simulink model "rotpentemplate"  (R2021b)
settings: Solver=ode45  StartTime=0.0  StopTime=100  RelTol=1e-3  EnableMultiTasking=on
values from neighbouring files (symbols this model uses):
  adingain = cfg.adingain    [hwinit.m]
  adinoffs = cfg.adinoffs    [hwinit.m]
  daoutgain = cfg.daoutgain    [hwinit.m]
  daoutoffs = cfg.daoutoffs    [hwinit.m]
  h = cfg.h    [hwinit.m]    (also in multisine.m = 0.005; prbs_signal.m = 0.001)
libraries: slpidlib x1
settings Model: Creator=rbabuska  LastModifiedBy=tsderksen
settings SolverCC: AlgebraicLoopSolver=TrustRegion
settings DataIOCC: LimitDataPoints=on  SaveFormat=Array  ReturnWorkspaceOutputs=off  SignalLoggingName=sigsOut
settings OptimizationCC: BooleanDataType=off  ExpressionDepthLimit=2147483647  InitFltsAndDblsToZero=on  LifeSpan=inf
settings DebuggingCC: SaveWithParameterizedLinksMsg=none  SignalResolutionControl=TryResolveAllWithWarning  MultiTaskDSMMsg=warning  MultiTaskCondExecSysMsg=none  AllowSymbolicDim=off  StateNameClashWarn=warning  SFUnexpectedBacktrackingDiag=warning  SFNoUnconditionalDefaultTransitionDiag=warning  SFExecutionAtInitializationDiag=none  SFMachineParentedDataDiag=warning  ArithmeticOperatorsInVariantConditions=warning
settings HardwareCC: ProdBitPerPointer=32  ProdBitPerSizeT=32  ProdBitPerPtrDiffT=32  ProdLargestAtomicFloat=None  ProdIntDivRoundTo=Undefined  ProdEndianess=Unspecified  ProdWordSize=32  ProdHWDeviceType=32-bit Generic  TargetUnknown=on
settings ModelReferenceCC: PropagateSignalLabelsOutOfModel=off
settings SFSimCC: SimUseLocalCustomCode=off  CustomCodeUndefinedFunction=UseInterfaceOnly
settings RTWCC: RTWUseLocalCustomCode=off
settings CodeAppCC: StateflowObjectComments=on
settings GRTTargetCC: TargetFcnLib=ansi_tfl_tmw.mat  TargetLangStandard=C89/C90 (ANSI)  CombineOutputUpdateFcns=off  GRTInterface=on
settings ConfigComp: CovMetricSettings=dw  CovSaveCumulativeToWorkspaceVar=on  CovSaveSingleToWorkspaceVar=on  CovExternalEMLEnable=off

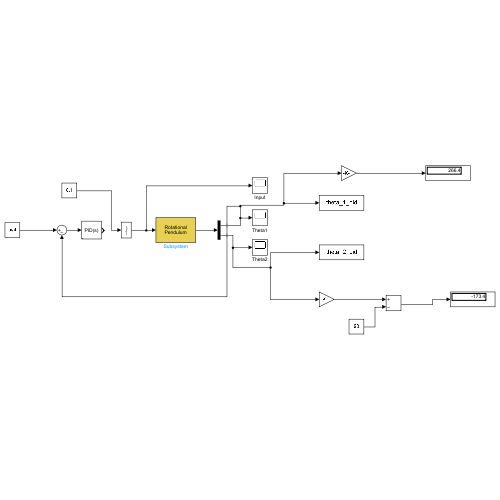
[thumbnail: Simulink's stored preview of the top-level diagram]
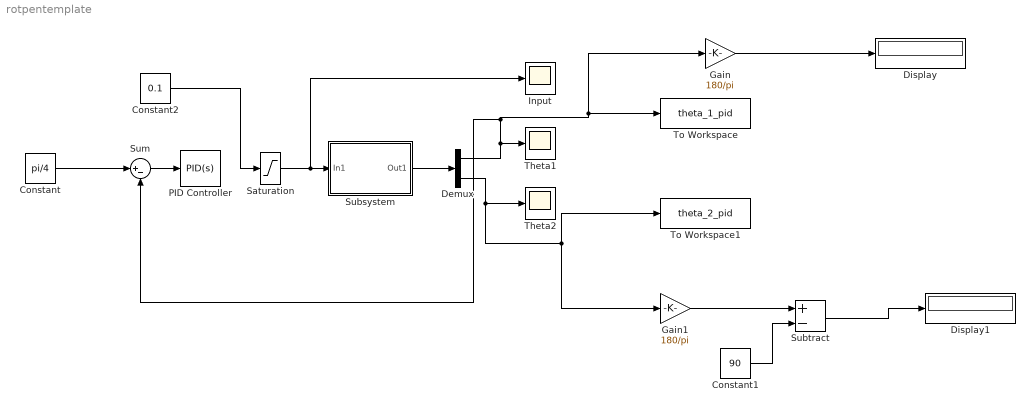
== system rotpentemplate ==
  Constant : Constant  Value=pi/4
  Constant1 : Constant  Value=90
  Constant2 : Constant  Value=0.1
  Demux : Demux  Outputs=2
  Display : Display
  Display1 : Display
  Gain : Gain  Gain=180/pi
  Gain1 : Gain  Gain=180/pi
  Input : Scope
  PID Controller : slpidlib/PID Controller  Controller=PID  Form=Parallel  TimeDomain=Continuous-time  UseExternalTs=off  SampleTime=-1  IntegratorMethod=Forward Euler  FilterMethod=Forward Euler  ControllerParametersSource=internal  P=0.1  I=0.1  D=0  UseFilter=on  N=100  TunerSelectOption=Transfer Function Based (PID Tuner App)  InitialConditionSource=internal  InitialConditionForIntegrator=0  InitialConditionForFilter=0  DifferentiatorICPrevScaledInput=0  ExternalReset=none  TrackingMode=off  Kt=1  LimitOutput=off  SatLimitsSource=internal  UpperSaturationLimit=inf  LowerSaturationLimit=-inf  LinearizeAsGain=on  AntiWindupMode=none  Kb=1  POutMin=[]  POutMax=[]  IOutMin=[]  IOutMax=[]  DOutMin=[]  DOutMax=[]  NOutMin=[]  NOutMax=[]  SumOutMin=[]  SumOutMax=[]  SaturationOutMin=[]  SaturationOutMax=[]  PParamMin=[]  PParamMax=[]  IParamMin=[]  IParamMax=[]  DParamMin=[]  DParamMax=[]  NParamMin=[]  NParamMax=[]  KbParamMin=[]  KbParamMax=[]  KtParamMin=[]  KtParamMax=[]  KbOutMin=[]  KbOutMax=[]  KtOutMin=[]  KtOutMax=[]  IntegratorOutMin=[]  IntegratorOutMax=[]  FilterOutMin=[]  FilterOutMax=[]  SumI1OutMin=[]  SumI1OutMax=[]  SumI2OutMin=[]  SumI2OutMax=[]  SumI3OutMin=[]  SumI3OutMax=[]  SumI4OutMin=[]  SumI4OutMax=[]  SumDOutMin=[]  SumDOutMax=[]  DifferentiatorOutMin=[]  DifferentiatorOutMax=[]  FilterDiffOutCoefMin=[]  FilterDiffOutCoefMax=[]  ReciprocalOutMin=[]  ReciprocalOutMax=[]  SumDenOutMin=[]  SumDenOutMax=[]  SumNumOutMin=[]  SumNumOutMax=[]  DivideOutMin=[]  DivideOutMax=[]  UdiffTsProdOutMin=[]  UdiffTsProdOutMax=[]  NTsProdOutMin=[]  NTsProdOutMax=[]  UintegralTsProdOutMin=[]  UintegralTsProdOutMax=[]  UngainTsProdOutMin=[]  UngainTsProdOutMax=[]  IntegratorContinuousStateAttributes=''  IntegratorStateMustResolveToSignalObject=off  IntegratorRTWStateStorageClass=Auto  FilterContinuousStateAttributes=''  FilterStateMustResolveToSignalObject=off  FilterRTWStateStorageClass=Auto  ParallelPVariant=InternalParameters  IdealPVariant=Disabled  IVariant=InternalParameters  DVariant=InternalParameters  IntegratorVariant=Continuous  SatVariant=Disabled  AWVariant=Passthrough  PCopyVariant=Disabled  TRVariant=Disabled  FdbkBlocksVariant=Forward  IdealPFdbkVariant=Disabled  SatFdbkVariant=Disabled  DerivativeFilterVariant=ContFilter  NVariant=InternalParameters  NCopyVariant=Disabled  FilterICVariant=InternalICsFilter  IntegratorICVariant=InternalICs  ExternalResetVariant=Disabled  TRSumVariant=Passthrough  SumFdbkVariant=Disabled  SumVariant=Sum_PID  TsampFilterVariant=InternalTs  TsampNgainVariant=Passthrough  TsampIntegralVariant=Passthrough  ExternalSaturationOutDataTypeStr=Inherit: Same as second input
  Saturation : Saturate  UpperLimit=1  LowerLimit=-1
  Subsystem : Subsystem
      mask Display: disp('Rotational\nPendulum')
  Subtract : Sum  Inputs=+-
  Sum : Sum  Inputs=|+-
  Theta1 : Scope
  Theta2 : Scope
  To Workspace : ToWorkspace  VariableName=theta_1_pid  SaveFormat=Timeseries  SampleTime=-1
  To Workspace1 : ToWorkspace  VariableName=theta_2_pid  SaveFormat=Timeseries  SampleTime=-1
  wires:
  Saturation/1 -> Subsystem/1(In1), Input/1
  Subsystem/1(Out1) -> Demux/1
  Demux/1 -> Theta1/1, Sum/2, To Workspace/1, Gain/1
  Demux/2 -> Theta2/1, Gain1/1, To Workspace1/1
  Constant1/1 -> Subtract/2
  Subtract/1 -> Display1/1
  Gain1/1 -> Subtract/1
  Gain/1 -> Display/1
  Constant/1 -> Sum/1
  Sum/1 -> PID Controller/1
  Constant2/1 -> Saturation/1

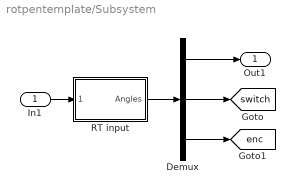
== system rotpentemplate/Subsystem ==
  In1 : Inport
  Demux : Demux  Outputs=[2 4 1]
  RT input : Subsystem  mask{Ts=h, channels=[6 7]}
      mask prompts: Ts "Sample time [s]:"; channels "Channels to read (e.g., [6 7])"
      mask init:
      | hwinit;
      | 
      | % initialize FPGA
      | fugihandle = fugiboard('Open', 'Pendulum1');
      | fugihandle.WatchdogTimeout = 0.5;
      | fugiboard('SetParams', fugihandle);
      | fugiboard('Write', fugihandle, 0, 0, 0, 0);  % dummy write to sync interface board
      | fugiboard('Write', fugihandle, 5, 1, 0, 0);  % reset position, activate relay
      | data = fugiboard('Read', fugihandle);        % get version info from FPGA
      | % model = bitshift(data(1), -5); 
      | % version = bitand(data(1), 31);
      | % disp(sprintf('FPGA setup %d, version %d', model, version)); % for the B&P it should say 1 1, or else there is a problem
      | fugiboard('Write', fugihandle, 0, 1, 0, 0);  % end reset
      | pause(0.1);                         % give relay some time to respond
      mask Display: disp('Rotational\nPendulum')
  Out1 : Outport
  tag scope: enc=global, switch=global
  wires:
  RT input/1(Angles) -> Demux/1
  Demux/1 -> Out1/1
  Demux/2 -> [switch]
  Demux/3 -> [enc]
  In1/1 -> RT input/1(Motors)

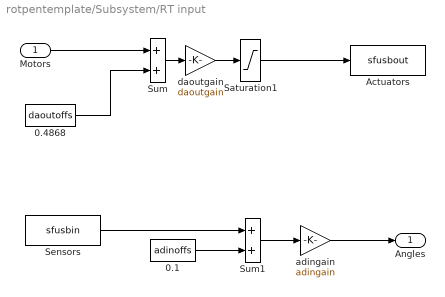
== system rotpentemplate/Subsystem/RT input ==
  Motors : Inport
  0.1 : Constant  Value=adinoffs
  0.4868 : Constant  Value=daoutoffs
  Actuators : S-Function  FunctionName=sfusbout  Parameters=Ts, fugihandle  SFunctionDeploymentMode=off  EnableBusSupport=off
  Saturation1 : Saturate  UpperLimit=10  LowerLimit=-10
  Sensors : S-Function  FunctionName=sfusbin  Parameters=Ts, fugihandle, channels  SFunctionDeploymentMode=off  EnableBusSupport=off
  Sum : Sum  InputSameDT=on  SaturateOnIntegerOverflow=on  OutDataTypeStr=Inherit: Same as first input
  Sum1 : Sum  InputSameDT=on  SaturateOnIntegerOverflow=on  OutDataTypeStr=Inherit: Same as first input
  adingain : Gain  Gain=adingain  SaturateOnIntegerOverflow=on  OutDataTypeStr=Inherit: Same as input  ParamDataTypeStr=Inherit: Same as input
  daoutgain : Gain  Gain=daoutgain  SaturateOnIntegerOverflow=on  OutDataTypeStr=Inherit: Same as input  ParamDataTypeStr=Inherit: Same as input
  Angles : Outport
  wires:
  Sum/1 -> daoutgain/1
  0.4868/1 -> Sum/2
  Motors/1 -> Sum/1
  Sum1/1 -> adingain/1
  0.1/1 -> Sum1/2
  adingain/1 -> Angles/1
  Saturation1/1 -> Actuators/1
  daoutgain/1 -> Saturation1/1
  Sensors/1 -> Sum1/1
